simulink model "traffic_LightModel"  (R2020a)
settings: Solver=VariableStepAuto  StartTime=0.0  StopTime=10.0  RelTol=1e-3
settings Model: Creator=INDRAJIT MARATHE  LastModifiedBy=INDRAJIT MARATHE

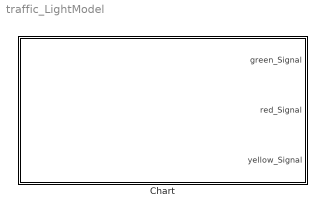
== system traffic_LightModel ==
  Chart : Stateflow chart  TreatAsAtomicUnit=on

== stateflow chart traffic_LightModel/Chart ==
  state go_Traffic
    en:
    green_Signal = 1;
    yellow_Signal=0;
    red_Signal=0;
  state stop_Traffic
    en:
    red_Signal=1;
    green_Signal = 0;
    yellow_Signal=0;
  state wait_Traffic
    en:
    yellow_Signal=1;
    green_Signal = 0;
    red_Signal=0;
  (default) -> stop_Traffic
  stop_Traffic -> go_Traffic : after(10,sec)
  wait_Traffic -> stop_Traffic : after(3,sec)
  go_Traffic -> wait_Traffic : after(5,sec)
  data: green_Signal output; red_Signal output; yellow_Signal output
